simulink model "eha_model_w_kf"  (R2015b)
settings: Solver=ode4  StartTime=0.0  StopTime=20  FixedStep=0.01  RelTol=1e-3
undefined symbols (not defined in the file): A, B, C, P0, x0
settings Model: Creator=mathi  LastModifiedBy=Nicholas

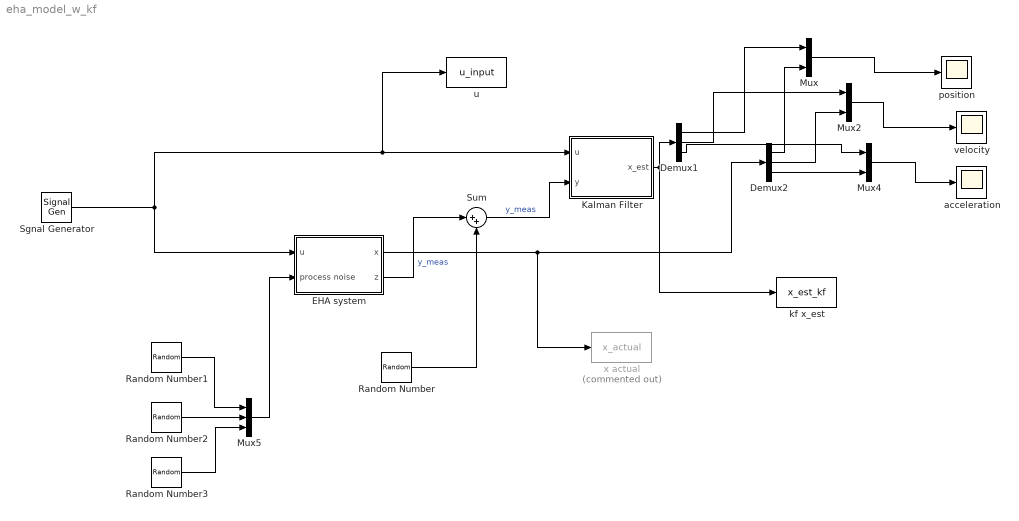
== system eha_model_w_kf ==
  Demux1 : Demux  Outputs=3
  Demux2 : Demux  Outputs=3
  EHA system : Subsystem
  Kalman Filter : Subsystem
  Mux : Mux  Inputs=2
  Mux2 : Mux  Inputs=2
  Mux4 : Mux  Inputs=2
  Mux5 : Mux  Inputs=3
  Random Number : RandomNumber  Variance=0.1  SampleTime=0.01
  Random Number1 : RandomNumber  Variance=0.01  SampleTime=0.01
  Random Number2 : RandomNumber  SampleTime=0.01
  Random Number3 : RandomNumber  Variance=10  SampleTime=0.01
  Sgnal Generator : SignalGenerator  WaveForm=square  Units=rad/sec
  Sum : Sum  Inputs=|++
  acceleration : Scope
  kf x_est : ToWorkspace  VariableName=x_est_kf  SaveFormat=Timeseries  SampleTime=-1
  position : Scope
  u : ToWorkspace  VariableName=u_input  SaveFormat=Timeseries  SampleTime=-1
  velocity : Scope
  x actual : ToWorkspace  Commented=on  VariableName=x_actual  SaveFormat=Timeseries  SampleTime=-1
  wires:
  Sgnal Generator/1 -> u/1, Kalman Filter/1(u), EHA system/1(u)
  EHA system/2(z) -> Sum/1  "y_meas"
  Sum/1 -> Kalman Filter/2(y)  "y_meas"
  Random Number/1 -> Sum/2
  Kalman Filter/1(x_est) -> Demux1/1, kf x_est/1
  EHA system/1(x) -> x actual/1, Demux2/1
  Demux1/1 -> Mux/1
  Demux2/1 -> Mux/2
  Mux/1 -> position/1
  Demux1/2 -> Mux2/1
  Demux2/2 -> Mux2/2
  Mux2/1 -> velocity/1
  Demux1/3 -> Mux4/1
  Demux2/3 -> Mux4/2
  Mux4/1 -> acceleration/1
  Random Number1/1 -> Mux5/1
  Random Number2/1 -> Mux5/2
  Random Number3/1 -> Mux5/3
  Mux5/1 -> EHA system/2(process noise)

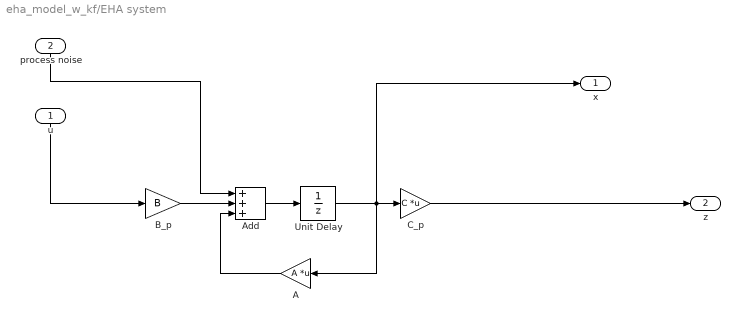
== system eha_model_w_kf/EHA system ==
  u : Inport
  process noise : Inport  Port=2
  A : Gain  Gain=A  Multiplication=Matrix(K*u)
  Add : Sum  Inputs=+++
  B_p : Gain  Gain=B
  C_p : Gain  Gain=C  Multiplication=Matrix(K*u)
  Unit Delay : UnitDelay  InitialCondition=x0  SampleTime=-1
  x : Outport
  z : Outport  Port=2
  wires:
  Unit Delay/1 -> C_p/1, x/1, A/1
  C_p/1 -> z/1
  u/1 -> B_p/1
  Add/1 -> Unit Delay/1
  B_p/1 -> Add/2
  A/1 -> Add/3
  process noise/1 -> Add/1

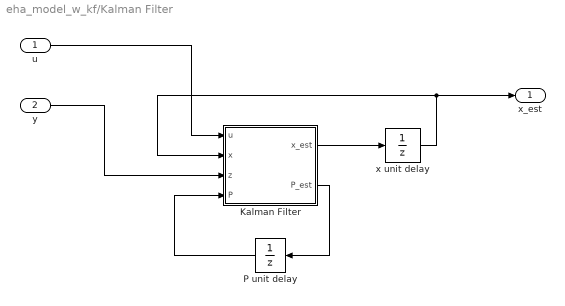
== system eha_model_w_kf/Kalman Filter ==
  u : Inport
  y : Inport  Port=2
  Kalman Filter : MATLAB Function  TreatAsAtomicUnit=on
  P unit delay : UnitDelay  InitialCondition=P0  SampleTime=-1
  x unit delay : UnitDelay  InitialCondition=x0  SampleTime=-1
  x_est : Outport
  wires:
  Kalman Filter/2(P_est) -> P unit delay/1
  Kalman Filter/1(x_est) -> x unit delay/1
  P unit delay/1 -> Kalman Filter/4(P)
  x unit delay/1 -> x_est/1, Kalman Filter/2(x)
  u/1 -> Kalman Filter/1(u)
  y/1 -> Kalman Filter/3(z)

== matlab function eha_model_w_kf/Kalman Filter/Kalman Filter ==
  data: u input; x_est output; x input; z input; P input; P_est output
function [x_est, P_est] = fcn(u,x,z,P)
%#codegen

A = [ 1 0.001 0; 0 1 0.001; -557.02 -28.616 0.9418];
B = [0 0 557.02]';
H = [1 0 0];
Q = 0.001*[ 1 0 0; 0 10 0; 0 0 100];
R = 10;
x_next = A*x + B*u;
P_next = A * P * A' + Q;


% Compute Kalman gain factor:
K_f =P*H'*pinv(H*P*H'+ R);
% Correction based on observation:
x_est = x_next + K_f*(z-H*x_next);
P_est = P_next - K_f*H*P_next;
